simulink model "LBR7_Duobot_ResolvedMotion"  (R2017b)
settings: Solver=ode1  StartTime=0.0  StopTime=12  FixedStep=0.001  RelTol=1e-3
PreLoadFcn:
  | Preload
values from neighbouring files (symbols this model uses):
  joint1_gain = 1    [Preload.m]    (also in PreloadTest.m)
  joint2_gain = 1    [Preload.m]    (also in PreloadTest.m)
  joint3_gain = 1    [Preload.m]    (also in PreloadTest.m)
  joint4_gain = 1    [Preload.m]    (also in PreloadTest.m)
  joint5_gain = 1    [Preload.m]    (also in PreloadTest.m)
  joint6_gain = 1    [Preload.m]    (also in PreloadTest.m)
  joint7_gain = 1    [Preload.m]    (also in PreloadTest.m)
  kuk = SerialLink(L)    [Preload.m]    (also in PreloadTest.m)
undefined symbols (not defined in the file or in its folder): jacky, X, Y, Z
libraries: sm_lib x154, nesl_utility x39
(part 1 of 4)
settings Model: Creator=jrv  LastModifiedBy=mkiri

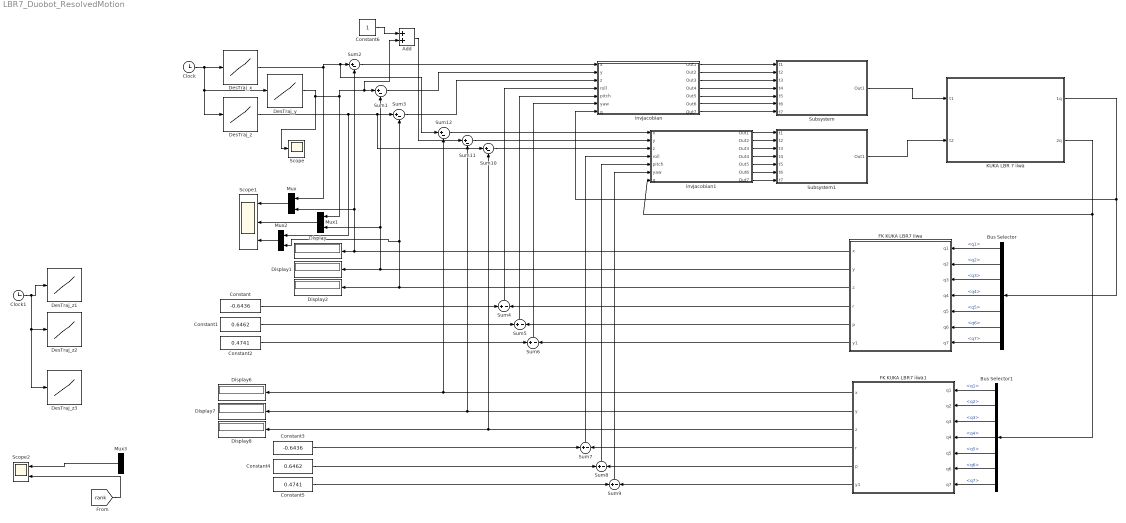
== system LBR7_Duobot_ResolvedMotion ==
  Add : Sum
  Bus Selector : BusSelector  OutputSignals=q1,q2,q3,q4,q5,q6,q7
  Bus Selector1 : BusSelector  OutputSignals=q1,q2,q3,q4,q5,q6,q7
  Clock : Clock
  Clock1 : Clock
  Constant : Constant  Value=-0.6436
  Constant1 : Constant  Value=0.6462
  Constant2 : Constant  Value=0.4741
  Constant3 : Constant  Value=-0.6436
  Constant4 : Constant  Value=0.6462
  Constant5 : Constant  Value=0.4741
  Constant6 : Constant
  DesTraj_x : Lookup_n-D  NumberOfTableDimensions=1  BreakpointsForDimension1=[0 5]  Table=[0.2314 0.2314]  ExtrapMethod=Clip  UseLastTableValue=on  InternalRulePriority=Speed  RndMeth=Simplest  InputSameDT=on
  DesTraj_y : Lookup_n-D  NumberOfTableDimensions=1  BreakpointsForDimension1=[0 12]  Table=[-0.2689 0.0689]  ExtrapMethod=Clip  UseLastTableValue=on  InternalRulePriority=Speed  RndMeth=Simplest  InputSameDT=on
  DesTraj_z : Lookup_n-D  NumberOfTableDimensions=1  BreakpointsForDimension1=[0 3 6 9 12]  Table=[0.9093 0.7093 0.9093 0.7093 0.9093]  InterpMethod=Cubic spline  ExtrapMethod=Clip  UseLastTableValue=on  InternalRulePriority=Speed  RndMeth=Simplest  InputSameDT=on
  DesTraj_z1 : Lookup_n-D  NumberOfTableDimensions=1  BreakpointsForDimension1=[0 1.5]  Table=[-0.6436 0]  ExtrapMethod=Clip  UseLastTableValue=on  InternalRulePriority=Speed  RndMeth=Simplest  InputSameDT=on
  DesTraj_z2 : Lookup_n-D  NumberOfTableDimensions=1  BreakpointsForDimension1=[0 1.5]  Table=[0.6462 0]  ExtrapMethod=Clip  UseLastTableValue=on  InternalRulePriority=Speed  RndMeth=Simplest  InputSameDT=on
  DesTraj_z3 : Lookup_n-D  NumberOfTableDimensions=1  BreakpointsForDimension1=[0 1.5]  Table=[0.4741 0]  ExtrapMethod=Clip  UseLastTableValue=on  InternalRulePriority=Speed  RndMeth=Simplest  InputSameDT=on
  Display{,1..2,6..8} (6 alike) : Display
  FK KUKA LBR7 iiwa : MATLAB Function  TreatAsAtomicUnit=on
  FK KUKA LBR7 iiwa1 : MATLAB Function  TreatAsAtomicUnit=on
  KUKA LBR 7 iiwa : Subsystem
  Mux : Mux  Inputs=2
  Mux1 : Mux  Inputs=2
  Mux2 : Mux  Inputs=2
  Mux3 : Mux  Inputs=3
  Scope : Scope
  Scope1 : Scope  NumInputPorts=3
  Scope2 : Scope  NumInputPorts=2
  Subsystem : Subsystem
  Subsystem1 : Subsystem
  Sum{1..3,10..12} (6 alike) : Sum  Inputs=|+-
  Sum{4..9} (6 alike) : Sum  Inputs=+-
  invJacobian : Subsystem
  invJacobian1 : Subsystem
  wires:
  Subsystem/1(Out1) -> KUKA LBR 7 iiwa/1(t1)
  KUKA LBR 7 iiwa/1(1q) -> invJacobian/7(q), Bus Selector/1
  Bus Selector/3 -> FK KUKA LBR7 iiwa/3(q3)  "<q3>"
  Bus Selector/2 -> FK KUKA LBR7 iiwa/2(q2)  "<q2>"
  Bus Selector/4 -> FK KUKA LBR7 iiwa/4(q4)  "<q4>"
  Bus Selector/1 -> FK KUKA LBR7 iiwa/1(q1)  "<q1>"
  Bus Selector/5 -> FK KUKA LBR7 iiwa/5(q5)  "<q5>"
  Bus Selector/6 -> FK KUKA LBR7 iiwa/6(q6)  "<q6>"
  Bus Selector/7 -> FK KUKA LBR7 iiwa/7(q7)  "<q7>"
  FK KUKA LBR7 iiwa/1(x) -> Mux/2, Sum2/2, Display/1
  FK KUKA LBR7 iiwa/2(y) -> Mux1/2, Sum1/2, Display1/1
  FK KUKA LBR7 iiwa/3(z) -> Mux2/2, Sum3/2, Display2/1
  DesTraj_x/1 -> Mux/1, Sum12/1, Sum2/1
  DesTraj_y/1 -> Scope/1, Mux1/1, Add/2, Sum1/1
  Sum2/1 -> invJacobian/1(x)
  Sum1/1 -> invJacobian/2(y)
  Sum3/1 -> invJacobian/3(z)
  DesTraj_z/1 -> Mux2/1, Sum10/1, Sum3/1
  invJacobian/1(Out1) -> Subsystem/1(t1)
  invJacobian/2(Out2) -> Subsystem/2(t2)
  invJacobian/3(Out3) -> Subsystem/3(t3)
  invJacobian/4(Out4) -> Subsystem/4(t4)
  invJacobian/5(Out5) -> Subsystem/5(t5)
  invJacobian/6(Out6) -> Subsystem/6(t6)
  invJacobian/7(Out7) -> Subsystem/7(t7)
  Clock/1 -> DesTraj_y/1, DesTraj_z/1, DesTraj_x/1
  Mux/1 -> Scope1/1
  Mux1/1 -> Scope1/2
  Mux2/1 -> Scope1/3
  FK KUKA LBR7 iiwa/4(r) -> Sum4/2
  FK KUKA LBR7 iiwa/5(p) -> Sum5/2
  Sum6/1 -> invJacobian/6(yaw)
  Sum4/1 -> invJacobian/4(roll)
  Mux3/1 -> Scope2/1
  [rank] -> Scope2/2
  Clock1/1 -> DesTraj_z3/1, DesTraj_z2/1, DesTraj_z1/1
  invJacobian1/7(Out7) -> Subsystem1/7(t7)
  invJacobian1/6(Out6) -> Subsystem1/6(t6)
  invJacobian1/5(Out5) -> Subsystem1/5(t5)
  invJacobian1/4(Out4) -> Subsystem1/4(t4)
  invJacobian1/3(Out3) -> Subsystem1/3(t3)
  invJacobian1/2(Out2) -> Subsystem1/2(t2)
  invJacobian1/1(Out1) -> Subsystem1/1(t1)
  Subsystem1/1(Out1) -> KUKA LBR 7 iiwa/2(t2)
  Bus Selector1/7 -> FK KUKA LBR7 iiwa1/7(q7)  "<q7>"
  Bus Selector1/6 -> FK KUKA LBR7 iiwa1/6(q6)  "<q6>"
  Bus Selector1/5 -> FK KUKA LBR7 iiwa1/5(q5)  "<q5>"
  Bus Selector1/1 -> FK KUKA LBR7 iiwa1/1(q1)  "<q1>"
  Bus Selector1/4 -> FK KUKA LBR7 iiwa1/4(q4)  "<q4>"
  Bus Selector1/2 -> FK KUKA LBR7 iiwa1/2(q2)  "<q2>"
  Bus Selector1/3 -> FK KUKA LBR7 iiwa1/3(q3)  "<q3>"
  KUKA LBR 7 iiwa/2(2q) -> Bus Selector1/1, invJacobian1/7(q)
  FK KUKA LBR7 iiwa1/1(x) -> Sum12/2, Display6/1
  FK KUKA LBR7 iiwa1/2(y) -> Sum11/2, Display7/1
  FK KUKA LBR7 iiwa1/3(z) -> Display8/1, Sum10/2
  Constant/1 -> Sum4/1
  Constant1/1 -> Sum5/1
  Constant2/1 -> Sum6/1
  FK KUKA LBR7 iiwa/6(y1) -> Sum6/2
  Sum5/1 -> invJacobian/5(pitch)
  Sum8/1 -> invJacobian1/5(pitch)
  FK KUKA LBR7 iiwa1/6(y1) -> Sum9/2
  Constant5/1 -> Sum9/1
  Constant4/1 -> Sum8/1
  Constant3/1 -> Sum7/1
  Sum7/1 -> invJacobian1/4(roll)
  Sum9/1 -> invJacobian1/6(yaw)
  FK KUKA LBR7 iiwa1/5(p) -> Sum8/2
  FK KUKA LBR7 iiwa1/4(r) -> Sum7/2
  Sum10/1 -> invJacobian1/3(z)
  Sum11/1 -> invJacobian1/2(y)
  Sum12/1 -> invJacobian1/1(x)
  Constant6/1 -> Add/1
  Add/1 -> Sum11/1

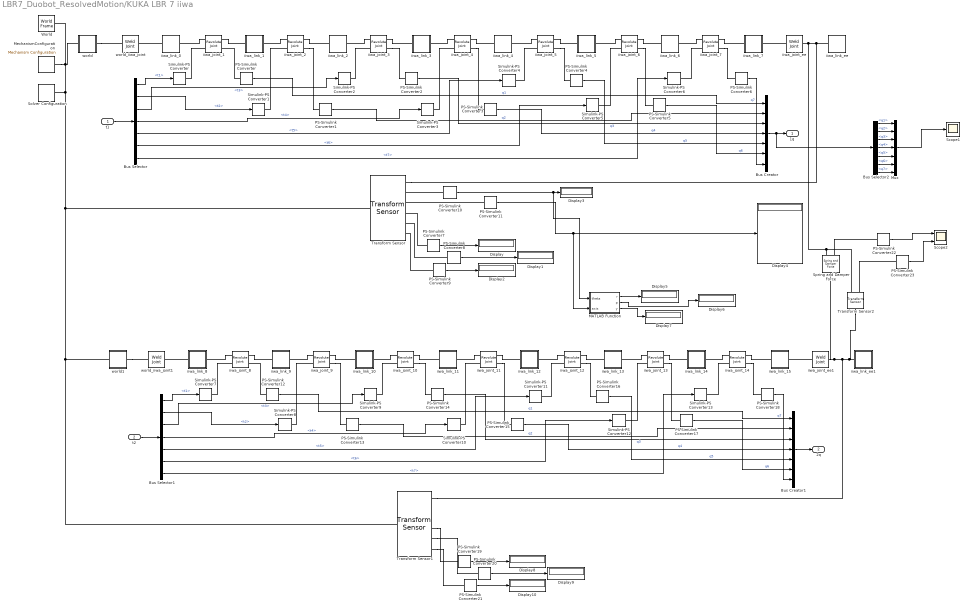
== system LBR7_Duobot_ResolvedMotion/KUKA LBR 7 iiwa ==
  t1 : Inport
  t2 : Inport  Port=2
  Bus Creator : BusCreator  Inputs=7
  Bus Creator1 : BusCreator  Inputs=7
  Bus Selector : BusSelector  OutputSignals=t1,t2,t3,t4,t5,t6,t7
  Bus Selector1 : BusSelector  OutputSignals=t1,t2,t3,t4,t5,t6,t7
  Bus Selector2 : BusSelector  OutputSignals=q1,q2,q3,q4,q5,q6,q7
  Display{,1..10} (11 alike) : Display
  MATLAB Function : MATLAB Function  TreatAsAtomicUnit=on
  MechanismConfiguration : sm_lib/Utilities/Mechanism Configuration  UniformGravity=Constant  GravityVector=[0 0 0]  GravityUnits=m/s^2  LinearizationDelta=0.001
  Mux : Mux  Inputs=7
  PS-Simulink Converter{,1..6,12..18} (14 alike) : nesl_utility/PS-Simulink Converter  PhysicalDomain=network_engine_domain  SubClassName=ps_output  LeftPortType=input  RightPortType=output  PseudoPeriodic=off  Frequencies=[]  Unit=rad  AffineConversion=off
  PS-Simulink Converter{7..11,19..21} (8 alike) : nesl_utility/PS-Simulink Converter  PhysicalDomain=network_engine_domain  SubClassName=ps_output  LeftPortType=input  RightPortType=output  PseudoPeriodic=off  Frequencies=[]  Unit=1  AffineConversion=off
  PS-Simulink Converter22 : nesl_utility/PS-Simulink Converter  PhysicalDomain=network_engine_domain  SubClassName=ps_output  LeftPortType=input  RightPortType=output  PseudoPeriodic=off  Frequencies=[]  Unit=N  AffineConversion=off
  PS-Simulink Converter23 : nesl_utility/PS-Simulink Converter  PhysicalDomain=network_engine_domain  SubClassName=ps_output  LeftPortType=input  RightPortType=output  PseudoPeriodic=off  Frequencies=[]  Unit=m  AffineConversion=off
  Scope1 : Scope
  Scope2 : Scope  NumInputPorts=2
  Simulink-PS Converter{,1..13} (14 alike) : nesl_utility/Simulink-PS Converter  PhysicalDomain=network_engine_domain  SubClassName=ps_input  LeftPortType=input  RightPortType=output  PseudoPeriodic=off  Frequencies=[]  NoiseDistribution=none  NoiseParameters=[]  Unit=N*m  AffineConversion=off  FilteringAndDerivatives=provide  SimscapeFilterOrder=1  InputFilterTimeConstant=0.001  UdotUserProvided=0
  Solver Configuration : nesl_utility/Solver Configuration  PhysicalDomain=network_engine_domain  SubClassName=solver  LeftPortType=input  RightPortType=generic  Accelerate=off  Tones=[]  Harmonics=[]  SimulateNoise=off  Profile=off  UseLocalSampling=off  EnableSwitchedLinearOptims=on  FrequencyDomain=off  UseCCode=off  RelTol=0.001  AbsTol=1e-06  MinStep=1e-09  ToWorkspace=off  RevertToSquareIcSolve=off  NumHomotopyIterations=100  PhasorMode=off  PhasorModeNumHarmonics=1  DoDC=off  ResidualTolerance=1e-09  UseLocalSolver=off  LocalSolverChoice=NE_BACKWARD_EULER_ADVANCER  LocalSolverSampleTime=0.001  DoFixedCost=off  MaxNonlinIter=3  MaxModeIter=2  LinearAlgebra=Sparse  DelaysMemoryBudget=1024  AutomaticFiltering=on  FilteringTimeConstant=0.001
  Spring and Damper Force : sm_lib/Forces and Torques/Spring and Damper Force  NaturalLength=1  NaturalLengthUnits=m  SpringStiffness=200000  SpringStiffnessUnits=N/m  DampingCoefficient=220  DampingCoefficientUnits=N/(m/s)  SenseForce=on
      settings: SourceProductName=Simscape Multibody
  Transform Sensor : sm_lib/Frames and Transforms/Transform Sensor  MeasurementFrame=World  SenseAngle=on  SenseAxis=on  SenseAngle1=off  SenseAngle2=off  SenseAngle3=off  SenseQ=off  SenseR=off  SenseOmegaX=off  SenseOmegaY=off  SenseOmegaZ=off  SenseOmega1=off  SenseOmega2=off  SenseOmega3=off  SenseQDot=off  SenseRDot=off  SenseAlphaX=off  SenseAlphaY=off  SenseAlphaZ=off  SenseAlpha1=off  SenseAlpha2=off  SenseAlpha3=off  SenseQDDot=off  SenseRDDot=off  SenseX=on  SenseY=on  SenseZ=on  SenseRad=off  SenseAzim=off  SenseDist=off  SenseInc=off  SenseXDot=off  SenseYDot=off  SenseZDot=off  SenseRadDot=off  SenseAzimDot=off  SenseDistDot=off  SenseIncDot=off  SenseXDDot=off  SenseYDDot=off  SenseZDDot=off  SenseRadDDot=off  SenseAzimDDot=off  SenseDistDDot=off  SenseIncDDot=off
  Transform Sensor1 : sm_lib/Frames and Transforms/Transform Sensor  MeasurementFrame=World  SenseAngle=on  SenseAxis=on  SenseAngle1=off  SenseAngle2=off  SenseAngle3=off  SenseQ=off  SenseR=off  SenseOmegaX=off  SenseOmegaY=off  SenseOmegaZ=off  SenseOmega1=off  SenseOmega2=off  SenseOmega3=off  SenseQDot=off  SenseRDot=off  SenseAlphaX=off  SenseAlphaY=off  SenseAlphaZ=off  SenseAlpha1=off  SenseAlpha2=off  SenseAlpha3=off  SenseQDDot=off  SenseRDDot=off  SenseX=on  SenseY=on  SenseZ=on  SenseRad=off  SenseAzim=off  SenseDist=off  SenseInc=off  SenseXDot=off  SenseYDot=off  SenseZDot=off  SenseRadDot=off  SenseAzimDot=off  SenseDistDot=off  SenseIncDot=off  SenseXDDot=off  SenseYDDot=off  SenseZDDot=off  SenseRadDDot=off  SenseAzimDDot=off  SenseDistDDot=off  SenseIncDDot=off
  Transform Sensor2 : sm_lib/Frames and Transforms/Transform Sensor  MeasurementFrame=World  SenseAngle=off  SenseAxis=off  SenseAngle1=off  SenseAngle2=off  SenseAngle3=off  SenseQ=off  SenseR=off  SenseOmegaX=off  SenseOmegaY=off  SenseOmegaZ=off  SenseOmega1=off  SenseOmega2=off  SenseOmega3=off  SenseQDot=off  SenseRDot=off  SenseAlphaX=off  SenseAlphaY=off  SenseAlphaZ=off  SenseAlpha1=off  SenseAlpha2=off  SenseAlpha3=off  SenseQDDot=off  SenseRDDot=off  SenseX=off  SenseY=off  SenseZ=off  SenseRad=off  SenseAzim=off  SenseDist=on  SenseInc=off  SenseXDot=off  SenseYDot=off  SenseZDot=off  SenseRadDot=off  SenseAzimDot=off  SenseDistDot=off  SenseIncDot=off  SenseXDDot=off  SenseYDDot=off  SenseZDDot=off  SenseRadDDot=off  SenseAzimDDot=off  SenseDistDDot=off  SenseIncDDot=off
  World : sm_lib/Frames and Transforms/World Frame
  iiwa_joint_1 : sm_lib/Joints/Revolute Joint  SenseConstraintForce=off  SenseConstraintForceX=off  SenseConstraintForceY=off  SenseConstraintForceZ=off  SenseConstraintTorque=off  SenseConstraintTorqueX=off  SenseConstraintTorqueY=off  SenseConstraintTorqueZ=off  SenseTotalForce=off  SenseTotalForceX=off  SenseTotalForceY=off  SenseTotalForceZ=off  SenseTotalTorque=off  SenseTotalTorqueX=off  SenseTotalTorqueY=off  SenseTotalTorqueZ=off  CompositeWrenchDir=FollowerOnBase  CompositeWrenchFrame=BaseFrame  EquilibriumPosition=0  EquilibriumPositionUnits=deg  SpringStiffness=0  SpringStiffnessUnits=N*m/deg  DampingCoefficient=0.5  DampingCoefficientUnits=m^2*kg/s/rad  TorqueActuationMode=InputTorque  MotionActuationMode=ComputedMotion  SensePosition=on  SenseVelocity=off  SenseAcceleration=off  SenseTorqueForce=off  PositionTargetSpecify=on  PositionTargetPriority=High  PositionTargetValue=joint1_initial_deg  PositionTargetValueUnits=deg  VelocityTargetSpecify=off  VelocityTargetPriority=High  VelocityTargetValue=0  VelocityTargetValueUnits=deg/s
  iiwa_joint_10 : sm_lib/Joints/Revolute Joint  SenseConstraintForce=off  SenseConstraintForceX=off  SenseConstraintForceY=off  SenseConstraintForceZ=off  SenseConstraintTorque=off  SenseConstraintTorqueX=off  SenseConstraintTorqueY=off  SenseConstraintTorqueZ=off  SenseTotalForce=off  SenseTotalForceX=off  SenseTotalForceY=off  SenseTotalForceZ=off  SenseTotalTorque=off  SenseTotalTorqueX=off  SenseTotalTorqueY=off  SenseTotalTorqueZ=off  CompositeWrenchDir=FollowerOnBase  CompositeWrenchFrame=BaseFrame  EquilibriumPosition=0  EquilibriumPositionUnits=deg  SpringStiffness=0  SpringStiffnessUnits=N*m/deg  DampingCoefficient=0.5  DampingCoefficientUnits=m^2*kg/s/rad  TorqueActuationMode=InputTorque  MotionActuationMode=ComputedMotion  SensePosition=on  SenseVelocity=off  SenseAcceleration=off  SenseTorqueForce=off  PositionTargetSpecify=on  PositionTargetPriority=High  PositionTargetValue=joint3_initial_deg2  PositionTargetValueUnits=deg  VelocityTargetSpecify=off  VelocityTargetPriority=High  VelocityTargetValue=0  VelocityTargetValueUnits=deg/s
  iiwa_joint_11 : sm_lib/Joints/Revolute Joint  SenseConstraintForce=off  SenseConstraintForceX=off  SenseConstraintForceY=off  SenseConstraintForceZ=off  SenseConstraintTorque=off  SenseConstraintTorqueX=off  SenseConstraintTorqueY=off  SenseConstraintTorqueZ=off  SenseTotalForce=off  SenseTotalForceX=off  SenseTotalForceY=off  SenseTotalForceZ=off  SenseTotalTorque=off  SenseTotalTorqueX=off  SenseTotalTorqueY=off  SenseTotalTorqueZ=off  CompositeWrenchDir=FollowerOnBase  CompositeWrenchFrame=BaseFrame  EquilibriumPosition=0  EquilibriumPositionUnits=deg  SpringStiffness=0  SpringStiffnessUnits=N*m/deg  DampingCoefficient=0.5  DampingCoefficientUnits=m^2*kg/s/rad  TorqueActuationMode=InputTorque  MotionActuationMode=ComputedMotion  SensePosition=on  SenseVelocity=off  SenseAcceleration=off  SenseTorqueForce=off  PositionTargetSpecify=on  PositionTargetPriority=High  PositionTargetValue=joint4_initial_deg2  PositionTargetValueUnits=deg  VelocityTargetSpecify=off  VelocityTargetPriority=High  VelocityTargetValue=0  VelocityTargetValueUnits=deg/s
  iiwa_joint_12 : sm_lib/Joints/Revolute Joint  SenseConstraintForce=off  SenseConstraintForceX=off  SenseConstraintForceY=off  SenseConstraintForceZ=off  SenseConstraintTorque=off  SenseConstraintTorqueX=off  SenseConstraintTorqueY=off  SenseConstraintTorqueZ=off  SenseTotalForce=off  SenseTotalForceX=off  SenseTotalForceY=off  SenseTotalForceZ=off  SenseTotalTorque=off  SenseTotalTorqueX=off  SenseTotalTorqueY=off  SenseTotalTorqueZ=off  CompositeWrenchDir=FollowerOnBase  CompositeWrenchFrame=BaseFrame  EquilibriumPosition=0  EquilibriumPositionUnits=deg  SpringStiffness=0  SpringStiffnessUnits=N*m/deg  DampingCoefficient=0.5  DampingCoefficientUnits=m^2*kg/s/rad  TorqueActuationMode=InputTorque  MotionActuationMode=ComputedMotion  SensePosition=on  SenseVelocity=off  SenseAcceleration=off  SenseTorqueForce=off  PositionTargetSpecify=on  PositionTargetPriority=High  PositionTargetValue=joint5_initial_deg2  PositionTargetValueUnits=deg  VelocityTargetSpecify=off  VelocityTargetPriority=High  VelocityTargetValue=0  VelocityTargetValueUnits=deg/s
  iiwa_joint_13 : sm_lib/Joints/Revolute Joint  SenseConstraintForce=off  SenseConstraintForceX=off  SenseConstraintForceY=off  SenseConstraintForceZ=off  SenseConstraintTorque=off  SenseConstraintTorqueX=off  SenseConstraintTorqueY=off  SenseConstraintTorqueZ=off  SenseTotalForce=off  SenseTotalForceX=off  SenseTotalForceY=off  SenseTotalForceZ=off  SenseTotalTorque=off  SenseTotalTorqueX=off  SenseTotalTorqueY=off  SenseTotalTorqueZ=off  CompositeWrenchDir=FollowerOnBase  CompositeWrenchFrame=BaseFrame  EquilibriumPosition=0  EquilibriumPositionUnits=deg  SpringStiffness=0  SpringStiffnessUnits=N*m/deg  DampingCoefficient=0.5  DampingCoefficientUnits=m^2*kg/s/rad  TorqueActuationMode=InputTorque  MotionActuationMode=ComputedMotion  SensePosition=on  SenseVelocity=off  SenseAcceleration=off  SenseTorqueForce=off  PositionTargetSpecify=on  PositionTargetPriority=High  PositionTargetValue=joint6_initial_deg2  PositionTargetValueUnits=deg  VelocityTargetSpecify=off  VelocityTargetPriority=High  VelocityTargetValue=0  VelocityTargetValueUnits=deg/s
  iiwa_joint_14 : sm_lib/Joints/Revolute Joint  SenseConstraintForce=off  SenseConstraintForceX=off  SenseConstraintForceY=off  SenseConstraintForceZ=off  SenseConstraintTorque=off  SenseConstraintTorqueX=off  SenseConstraintTorqueY=off  SenseConstraintTorqueZ=off  SenseTotalForce=off  SenseTotalForceX=off  SenseTotalForceY=off  SenseTotalForceZ=off  SenseTotalTorque=off  SenseTotalTorqueX=off  SenseTotalTorqueY=off  SenseTotalTorqueZ=off  CompositeWrenchDir=FollowerOnBase  CompositeWrenchFrame=BaseFrame  EquilibriumPosition=0  EquilibriumPositionUnits=deg  SpringStiffness=0  SpringStiffnessUnits=N*m/deg  DampingCoefficient=0.5  DampingCoefficientUnits=m^2*kg/s/rad  TorqueActuationMode=InputTorque  MotionActuationMode=ComputedMotion  SensePosition=on  SenseVelocity=off  SenseAcceleration=off  SenseTorqueForce=off  PositionTargetSpecify=on  PositionTargetPriority=High  PositionTargetValue=joint7_initial_deg2  PositionTargetValueUnits=deg  VelocityTargetSpecify=off  VelocityTargetPriority=High  VelocityTargetValue=0  VelocityTargetValueUnits=deg/s
  iiwa_joint_2 : sm_lib/Joints/Revolute Joint  SenseConstraintForce=off  SenseConstraintForceX=off  SenseConstraintForceY=off  SenseConstraintForceZ=off  SenseConstraintTorque=off  SenseConstraintTorqueX=off  SenseConstraintTorqueY=off  SenseConstraintTorqueZ=off  SenseTotalForce=off  SenseTotalForceX=off  SenseTotalForceY=off  SenseTotalForceZ=off  SenseTotalTorque=off  SenseTotalTorqueX=off  SenseTotalTorqueY=off  SenseTotalTorqueZ=off  CompositeWrenchDir=FollowerOnBase  CompositeWrenchFrame=BaseFrame  EquilibriumPosition=0  EquilibriumPositionUnits=deg  SpringStiffness=0  SpringStiffnessUnits=N*m/deg  DampingCoefficient=0.5  DampingCoefficientUnits=m^2*kg/s/rad  TorqueActuationMode=InputTorque  MotionActuationMode=ComputedMotion  SensePosition=on  SenseVelocity=off  SenseAcceleration=off  SenseTorqueForce=off  PositionTargetSpecify=on  PositionTargetPriority=High  PositionTargetValue=joint2_initial_deg  PositionTargetValueUnits=deg  VelocityTargetSpecify=off  VelocityTargetPriority=High  VelocityTargetValue=0  VelocityTargetValueUnits=deg/s
  iiwa_joint_3 : sm_lib/Joints/Revolute Joint  SenseConstraintForce=off  SenseConstraintForceX=off  SenseConstraintForceY=off  SenseConstraintForceZ=off  SenseConstraintTorque=off  SenseConstraintTorqueX=off  SenseConstraintTorqueY=off  SenseConstraintTorqueZ=off  SenseTotalForce=off  SenseTotalForceX=off  SenseTotalForceY=off  SenseTotalForceZ=off  SenseTotalTorque=off  SenseTotalTorqueX=off  SenseTotalTorqueY=off  SenseTotalTorqueZ=off  CompositeWrenchDir=FollowerOnBase  CompositeWrenchFrame=BaseFrame  EquilibriumPosition=0  EquilibriumPositionUnits=deg  SpringStiffness=0  SpringStiffnessUnits=N*m/deg  DampingCoefficient=0.5  DampingCoefficientUnits=m^2*kg/s/rad  TorqueActuationMode=InputTorque  MotionActuationMode=ComputedMotion  SensePosition=on  SenseVelocity=off  SenseAcceleration=off  SenseTorqueForce=off  PositionTargetSpecify=on  PositionTargetPriority=High  PositionTargetValue=joint3_initial_deg  PositionTargetValueUnits=deg  VelocityTargetSpecify=off  VelocityTargetPriority=High  VelocityTargetValue=0  VelocityTargetValueUnits=deg/s
  iiwa_joint_4 : sm_lib/Joints/Revolute Joint  SenseConstraintForce=off  SenseConstraintForceX=off  SenseConstraintForceY=off  SenseConstraintForceZ=off  SenseConstraintTorque=off  SenseConstraintTorqueX=off  SenseConstraintTorqueY=off  SenseConstraintTorqueZ=off  SenseTotalForce=off  SenseTotalForceX=off  SenseTotalForceY=off  SenseTotalForceZ=off  SenseTotalTorque=off  SenseTotalTorqueX=off  SenseTotalTorqueY=off  SenseTotalTorqueZ=off  CompositeWrenchDir=FollowerOnBase  CompositeWrenchFrame=BaseFrame  EquilibriumPosition=0  EquilibriumPositionUnits=deg  SpringStiffness=0  SpringStiffnessUnits=N*m/deg  DampingCoefficient=0.5  DampingCoefficientUnits=m^2*kg/s/rad  TorqueActuationMode=InputTorque  MotionActuationMode=ComputedMotion  SensePosition=on  SenseVelocity=off  SenseAcceleration=off  SenseTorqueForce=off  PositionTargetSpecify=on  PositionTargetPriority=High  PositionTargetValue=joint4_initial_deg  PositionTargetValueUnits=deg  VelocityTargetSpecify=off  VelocityTargetPriority=High  VelocityTargetValue=0  VelocityTargetValueUnits=deg/s
  iiwa_joint_5 : sm_lib/Joints/Revolute Joint  SenseConstraintForce=off  SenseConstraintForceX=off  SenseConstraintForceY=off  SenseConstraintForceZ=off  SenseConstraintTorque=off  SenseConstraintTorqueX=off  SenseConstraintTorqueY=off  SenseConstraintTorqueZ=off  SenseTotalForce=off  SenseTotalForceX=off  SenseTotalForceY=off  SenseTotalForceZ=off  SenseTotalTorque=off  SenseTotalTorqueX=off  SenseTotalTorqueY=off  SenseTotalTorqueZ=off  CompositeWrenchDir=FollowerOnBase  CompositeWrenchFrame=BaseFrame  EquilibriumPosition=0  EquilibriumPositionUnits=deg  SpringStiffness=0  SpringStiffnessUnits=N*m/deg  DampingCoefficient=0.5  DampingCoefficientUnits=m^2*kg/s/rad  TorqueActuationMode=InputTorque  MotionActuationMode=ComputedMotion  SensePosition=on  SenseVelocity=off  SenseAcceleration=off  SenseTorqueForce=off  PositionTargetSpecify=on  PositionTargetPriority=High  PositionTargetValue=joint5_initial_deg  PositionTargetValueUnits=deg  VelocityTargetSpecify=off  VelocityTargetPriority=High  VelocityTargetValue=0  VelocityTargetValueUnits=deg/s
  iiwa_joint_6 : sm_lib/Joints/Revolute Joint  SenseConstraintForce=off  SenseConstraintForceX=off  SenseConstraintForceY=off  SenseConstraintForceZ=off  SenseConstraintTorque=off  SenseConstraintTorqueX=off  SenseConstraintTorqueY=off  SenseConstraintTorqueZ=off  SenseTotalForce=off  SenseTotalForceX=off  SenseTotalForceY=off  SenseTotalForceZ=off  SenseTotalTorque=off  SenseTotalTorqueX=off  SenseTotalTorqueY=off  SenseTotalTorqueZ=off  CompositeWrenchDir=FollowerOnBase  CompositeWrenchFrame=BaseFrame  EquilibriumPosition=0  EquilibriumPositionUnits=deg  SpringStiffness=0  SpringStiffnessUnits=N*m/deg  DampingCoefficient=0.5  DampingCoefficientUnits=m^2*kg/s/rad  TorqueActuationMode=InputTorque  MotionActuationMode=ComputedMotion  SensePosition=on  SenseVelocity=off  SenseAcceleration=off  SenseTorqueForce=off  PositionTargetSpecify=on  PositionTargetPriority=High  PositionTargetValue=joint6_initial_deg  PositionTargetValueUnits=deg  VelocityTargetSpecify=off  VelocityTargetPriority=High  VelocityTargetValue=0  VelocityTargetValueUnits=deg/s
  iiwa_joint_7 : sm_lib/Joints/Revolute Joint  SenseConstraintForce=off  SenseConstraintForceX=off  SenseConstraintForceY=off  SenseConstraintForceZ=off  SenseConstraintTorque=off  SenseConstraintTorqueX=off  SenseConstraintTorqueY=off  SenseConstraintTorqueZ=off  SenseTotalForce=off  SenseTotalForceX=off  SenseTotalForceY=off  SenseTotalForceZ=off  SenseTotalTorque=off  SenseTotalTorqueX=off  SenseTotalTorqueY=off  SenseTotalTorqueZ=off  CompositeWrenchDir=FollowerOnBase  CompositeWrenchFrame=BaseFrame  EquilibriumPosition=0  EquilibriumPositionUnits=deg  SpringStiffness=0  SpringStiffnessUnits=N*m/deg  DampingCoefficient=0.5  DampingCoefficientUnits=m^2*kg/s/rad  TorqueActuationMode=InputTorque  MotionActuationMode=ComputedMotion  SensePosition=on  SenseVelocity=off  SenseAcceleration=off  SenseTorqueForce=off  PositionTargetSpecify=on  PositionTargetPriority=High  PositionTargetValue=joint7_initial_deg  PositionTargetValueUnits=deg  VelocityTargetSpecify=off  VelocityTargetPriority=High  VelocityTargetValue=0  VelocityTargetValueUnits=deg/s
  iiwa_joint_8 : sm_lib/Joints/Revolute Joint  SenseConstraintForce=off  SenseConstraintForceX=off  SenseConstraintForceY=off  SenseConstraintForceZ=off  SenseConstraintTorque=off  SenseConstraintTorqueX=off  SenseConstraintTorqueY=off  SenseConstraintTorqueZ=off  SenseTotalForce=off  SenseTotalForceX=off  SenseTotalForceY=off  SenseTotalForceZ=off  SenseTotalTorque=off  SenseTotalTorqueX=off  SenseTotalTorqueY=off  SenseTotalTorqueZ=off  CompositeWrenchDir=FollowerOnBase  CompositeWrenchFrame=BaseFrame  EquilibriumPosition=0  EquilibriumPositionUnits=deg  SpringStiffness=0  SpringStiffnessUnits=N*m/deg  DampingCoefficient=0.5  DampingCoefficientUnits=m^2*kg/s/rad  TorqueActuationMode=InputTorque  MotionActuationMode=ComputedMotion  SensePosition=on  SenseVelocity=off  SenseAcceleration=off  SenseTorqueForce=off  PositionTargetSpecify=on  PositionTargetPriority=High  PositionTargetValue=joint1_initial_deg2  PositionTargetValueUnits=deg  VelocityTargetSpecify=off  VelocityTargetPriority=High  VelocityTargetValue=0  VelocityTargetValueUnits=deg/s
  iiwa_joint_9 : sm_lib/Joints/Revolute Joint  SenseConstraintForce=off  SenseConstraintForceX=off  SenseConstraintForceY=off  SenseConstraintForceZ=off  SenseConstraintTorque=off  SenseConstraintTorqueX=off  SenseConstraintTorqueY=off  SenseConstraintTorqueZ=off  SenseTotalForce=off  SenseTotalForceX=off  SenseTotalForceY=off  SenseTotalForceZ=off  SenseTotalTorque=off  SenseTotalTorqueX=off  SenseTotalTorqueY=off  SenseTotalTorqueZ=off  CompositeWrenchDir=FollowerOnBase  CompositeWrenchFrame=BaseFrame  EquilibriumPosition=0  EquilibriumPositionUnits=deg  SpringStiffness=0  SpringStiffnessUnits=N*m/deg  DampingCoefficient=0.5  DampingCoefficientUnits=m^2*kg/s/rad  TorqueActuationMode=InputTorque  MotionActuationMode=ComputedMotion  SensePosition=on  SenseVelocity=off  SenseAcceleration=off  SenseTorqueForce=off  PositionTargetSpecify=on  PositionTargetPriority=High  PositionTargetValue=joint2_initial_deg2  PositionTargetValueUnits=deg  VelocityTargetSpecify=off  VelocityTargetPriority=High  VelocityTargetValue=0  VelocityTargetValueUnits=deg/s
  iiwa_joint_ee : sm_lib/Joints/Weld Joint  SenseConstraintForce=off  SenseConstraintForceX=off  SenseConstraintForceY=off  SenseConstraintForceZ=off  SenseConstraintTorque=off  SenseConstraintTorqueX=off  SenseConstraintTorqueY=off  SenseConstraintTorqueZ=off  SenseTotalForce=off  SenseTotalForceX=off  SenseTotalForceY=off  SenseTotalForceZ=off  SenseTotalTorque=off  SenseTotalTorqueX=off  SenseTotalTorqueY=off  SenseTotalTorqueZ=off  CompositeWrenchDir=FollowerOnBase  CompositeWrenchFrame=BaseFrame
  iiwa_joint_ee1 : sm_lib/Joints/Weld Joint  SenseConstraintForce=off  SenseConstraintForceX=off  SenseConstraintForceY=off  SenseConstraintForceZ=off  SenseConstraintTorque=off  SenseConstraintTorqueX=off  SenseConstraintTorqueY=off  SenseConstraintTorqueZ=off  SenseTotalForce=off  SenseTotalForceX=off  SenseTotalForceY=off  SenseTotalForceZ=off  SenseTotalTorque=off  SenseTotalTorqueX=off  SenseTotalTorqueY=off  SenseTotalTorqueZ=off  CompositeWrenchDir=FollowerOnBase  CompositeWrenchFrame=BaseFrame
  iiwa_link_0 : Subsystem
  iiwa_link_1 : Subsystem
  iiwa_link_10 : Subsystem
  iiwa_link_11 : Subsystem
  iiwa_link_12 : Subsystem
  iiwa_link_13 : Subsystem
  iiwa_link_14 : Subsystem
  iiwa_link_15 : Subsystem
  iiwa_link_2 : Subsystem
  iiwa_link_3 : Subsystem
  iiwa_link_4 : Subsystem
  iiwa_link_5 : Subsystem
  iiwa_link_6 : Subsystem
  iiwa_link_7 : Subsystem
  iiwa_link_8 : Subsystem
  iiwa_link_9 : Subsystem
  iiwa_link_ee : Subsystem
  iiwa_link_ee1 : Subsystem
  world : Subsystem
  world1 : Subsystem
  world_iiwa_joint : sm_lib/Joints/Weld Joint  SenseConstraintForce=off  SenseConstraintForceX=off  SenseConstraintForceY=off  SenseConstraintForceZ=off  SenseConstraintTorque=off  SenseConstraintTorqueX=off  SenseConstraintTorqueY=off  SenseConstraintTorqueZ=off  SenseTotalForce=off  SenseTotalForceX=off  SenseTotalForceY=off  SenseTotalForceZ=off  SenseTotalTorque=off  SenseTotalTorqueX=off  SenseTotalTorqueY=off  SenseTotalTorqueZ=off  CompositeWrenchDir=FollowerOnBase  CompositeWrenchFrame=BaseFrame
  world_iiwa_joint1 : sm_lib/Joints/Weld Joint  SenseConstraintForce=off  SenseConstraintForceX=off  SenseConstraintForceY=off  SenseConstraintForceZ=off  SenseConstraintTorque=off  SenseConstraintTorqueX=off  SenseConstraintTorqueY=off  SenseConstraintTorqueZ=off  SenseTotalForce=off  SenseTotalForceX=off  SenseTotalForceY=off  SenseTotalForceZ=off  SenseTotalTorque=off  SenseTotalTorqueX=off  SenseTotalTorqueY=off  SenseTotalTorqueZ=off  CompositeWrenchDir=FollowerOnBase  CompositeWrenchFrame=BaseFrame
  1q : Outport
  2q : Outport  Port=2
  wires:
  PS-Simulink Converter7/1 -> Display/1
  PS-Simulink Converter9/1 -> Display2/1
  PS-Simulink Converter8/1 -> Display1/1
  PS-Simulink Converter/1 -> Bus Creator/1  "q1"
  PS-Simulink Converter1/1 -> Bus Creator/2  "q2"
  PS-Simulink Converter2/1 -> Bus Creator/3  "q3"
  PS-Simulink Converter3/1 -> Bus Creator/4  "q4"
  PS-Simulink Converter4/1 -> Bus Creator/5  "q5"
  PS-Simulink Converter5/1 -> Bus Creator/6  "q6"
  PS-Simulink Converter6/1 -> Bus Creator/7  "q7"
  t1/1 -> Bus Selector/1
  Bus Selector/1 -> Simulink-PS Converter/1  "<t1>"
  Bus Selector/2 -> Simulink-PS Converter1/1  "<t2>"
  Bus Selector/3 -> Simulink-PS Converter2/1  "<t3>"
  Bus Selector/4 -> Simulink-PS Converter3/1  "<t4>"
  Bus Selector/5 -> Simulink-PS Converter4/1  "<t5>"
  Bus Selector/6 -> Simulink-PS Converter5/1  "<t6>"
  Bus Selector/7 -> Simulink-PS Converter6/1  "<t7>"
  PS-Simulink Converter10/1 -> MATLAB Function/1(theta), Display3/1
  PS-Simulink Converter11/1 -> MATLAB Function/2(axis), Display4/1
  MATLAB Function/1(r) -> Display5/1
  MATLAB Function/3(y) -> Display7/1
  MATLAB Function/2(p) -> Display6/1
  Bus Selector1/7 -> Simulink-PS Converter13/1  "<t7>"
  Bus Selector1/6 -> Simulink-PS Converter12/1  "<t6>"
  Bus Selector1/5 -> Simulink-PS Converter11/1  "<t5>"
  Bus Selector1/4 -> Simulink-PS Converter10/1  "<t4>"
  Bus Selector1/3 -> Simulink-PS Converter9/1  "<t3>"
  Bus Selector1/2 -> Simulink-PS Converter8/1  "<t2>"
  Bus Selector1/1 -> Simulink-PS Converter7/1  "<t1>"
  t2/1 -> Bus Selector1/1
  Bus Creator1/1 -> 2q/1
  PS-Simulink Converter18/1 -> Bus Creator1/7  "q7"
  PS-Simulink Converter17/1 -> Bus Creator1/6  "q6"
  PS-Simulink Converter16/1 -> Bus Creator1/5  "q5"
  PS-Simulink Converter15/1 -> Bus Creator1/4  "q4"
  PS-Simulink Converter14/1 -> Bus Creator1/3  "q3"
  PS-Simulink Converter13/1 -> Bus Creator1/2  "q2"
  PS-Simulink Converter12/1 -> Bus Creator1/1  "q1"
  PS-Simulink Converter20/1 -> Display9/1
  PS-Simulink Converter21/1 -> Display10/1
  PS-Simulink Converter19/1 -> Display8/1
  PS-Simulink Converter22/1 -> Scope2/1
  PS-Simulink Converter23/1 -> Scope2/2
  Bus Creator/1 -> Bus Selector2/1, 1q/1
  Bus Selector2/1 -> Mux/1  "<q1>"
  Mux/1 -> Scope1/1
  Bus Selector2/6 -> Mux/6  "<q6>"
  Bus Selector2/2 -> Mux/2  "<q2>"
  Bus Selector2/3 -> Mux/3  "<q3>"
  Bus Selector2/5 -> Mux/5  "<q5>"
  Bus Selector2/7 -> Mux/7  "<q7>"
  Bus Selector2/4 -> Mux/4  "<q4>"
  connections:
  Simulink-PS Converter/RConn1 -- iiwa_joint_1/LConn2
  iiwa_joint_5/RConn2 -- PS-Simulink Converter4/LConn1
  iiwa_joint_5/LConn2 -- Simulink-PS Converter4/RConn1
  PS-Simulink Converter/LConn1 -- iiwa_joint_1/RConn2
  iiwa_joint_2/LConn2 -- Simulink-PS Converter1/RConn1
  iiwa_joint_2/RConn2 -- PS-Simulink Converter1/LConn1
  iiwa_joint_6/RConn2 -- PS-Simulink Converter5/LConn1
  iiwa_joint_6/LConn2 -- Simulink-PS Converter5/RConn1
  iiwa_joint_7/RConn2 -- PS-Simulink Converter6/LConn1
  iiwa_joint_7/LConn2 -- Simulink-PS Converter6/RConn1
  iiwa_joint_1/LConn1 -- iiwa_link_0/RConn1
  iiwa_joint_ee/LConn1 -- iiwa_link_7/RConn1
  iiwa_joint_2/RConn1 -- iiwa_link_2/LConn1
  iiwa_joint_7/RConn1 -- iiwa_link_7/LConn1
  iiwa_link_0/LConn1 -- world_iiwa_joint/RConn1
  iiwa_joint_6/RConn1 -- iiwa_link_6/LConn1
  world/RConn1 -- world_iiwa_joint/LConn1
  iiwa_joint_3/RConn1 -- iiwa_link_3/LConn1
  iiwa_joint_4/LConn1 -- iiwa_link_3/RConn1
  World/RConn1 -- Transform Sensor1/LConn1 -- world1/LConn1 -- Transform Sensor/LConn1 -- Solver Configuration/RConn1 -- MechanismConfiguration/RConn1 -- world/LConn1
  iiwa_joint_6/LConn1 -- iiwa_link_5/RConn1
  iiwa_joint_3/LConn1 -- iiwa_link_2/RConn1
  iiwa_joint_5/RConn1 -- iiwa_link_5/LConn1
  iiwa_joint_5/LConn1 -- iiwa_link_4/RConn1
  iiwa_joint_ee/RConn1 -- Transform Sensor2/RConn1 -- Spring and Damper Force/RConn1 -- iiwa_link_ee/LConn1 -- Transform Sensor/RConn1
  iiwa_joint_2/LConn1 -- iiwa_link_1/RConn1
  iiwa_joint_7/LConn1 -- iiwa_link_6/RConn1
  iiwa_joint_1/RConn1 -- iiwa_link_1/LConn1
  iiwa_joint_4/RConn1 -- iiwa_link_4/LConn1
  iiwa_joint_4/LConn2 -- Simulink-PS Converter3/RConn1
  iiwa_joint_4/RConn2 -- PS-Simulink Converter3/LConn1
  iiwa_joint_3/RConn2 -- PS-Simulink Converter2/LConn1
  iiwa_joint_3/LConn2 -- Simulink-PS Converter2/RConn1
  PS-Simulink Converter10/LConn1 -- Transform Sensor/RConn2
  PS-Simulink Converter11/LConn1 -- Transform Sensor/RConn3
  PS-Simulink Converter7/LConn1 -- Transform Sensor/RConn4
  PS-Simulink Converter9/LConn1 -- Transform Sensor/RConn6
  PS-Simulink Converter8/LConn1 -- Transform Sensor/RConn5
  iiwa_joint_ee1/RConn1 -- Transform Sensor2/LConn1 -- iiwa_link_ee1/LConn1 -- Transform Sensor1/RConn1 -- Spring and Damper Force/LConn1
  iiwa_joint_10/RConn2 -- PS-Simulink Converter14/LConn1
  iiwa_joint_11/RConn2 -- PS-Simulink Converter15/LConn1
  iiwa_joint_11/RConn1 -- iiwa_link_12/LConn1
  iiwa_joint_14/LConn1 -- iiwa_link_14/RConn1
  iiwa_joint_12/LConn1 -- iiwa_link_12/RConn1
  iiwa_joint_10/LConn1 -- iiwa_link_10/RConn1
  iiwa_joint_12/RConn1 -- iiwa_link_13/LConn1
  iiwa_joint_13/LConn1 -- iiwa_link_13/RConn1
  iiwa_joint_11/LConn1 -- iiwa_link_11/RConn1
  iiwa_joint_10/RConn1 -- iiwa_link_11/LConn1
  iiwa_joint_9/LConn1 -- iiwa_link_9/RConn1
  world1/RConn1 -- world_iiwa_joint1/LConn1
  iiwa_joint_13/RConn1 -- iiwa_link_14/LConn1
  iiwa_joint_14/RConn1 -- iiwa_link_15/LConn1
  iiwa_joint_9/RConn1 -- iiwa_link_10/LConn1
  iiwa_joint_11/LConn2 -- Simulink-PS Converter10/RConn1
  iiwa_joint_ee1/LConn1 -- iiwa_link_15/RConn1
  iiwa_joint_14/LConn2 -- Simulink-PS Converter13/RConn1
  iiwa_joint_8/LConn1 -- iiwa_link_8/RConn1
  iiwa_joint_14/RConn2 -- PS-Simulink Converter18/LConn1
  iiwa_joint_13/RConn2 -- PS-Simulink Converter17/LConn1
  iiwa_link_8/LConn1 -- world_iiwa_joint1/RConn1
  iiwa_joint_13/LConn2 -- Simulink-PS Converter12/RConn1
  iiwa_joint_9/RConn2 -- PS-Simulink Converter13/LConn1
  iiwa_joint_8/RConn1 -- iiwa_link_9/LConn1
  iiwa_joint_12/LConn2 -- Simulink-PS Converter11/RConn1
  iiwa_joint_10/LConn2 -- Simulink-PS Converter9/RConn1
  iiwa_joint_12/RConn2 -- PS-Simulink Converter16/LConn1
  iiwa_joint_9/LConn2 -- Simulink-PS Converter8/RConn1
  Simulink-PS Converter7/RConn1 -- iiwa_joint_8/LConn2
  PS-Simulink Converter12/LConn1 -- iiwa_joint_8/RConn2
  Transform Sensor1/RConn5 -- PS-Simulink Converter20/LConn1
  Transform Sensor1/RConn6 -- PS-Simulink Converter21/LConn1
  Transform Sensor1/RConn4 -- PS-Simulink Converter19/LConn1
  PS-Simulink Converter22/LConn1 -- Spring and Damper Force/RConn2
  PS-Simulink Converter23/LConn1 -- Transform Sensor2/RConn2

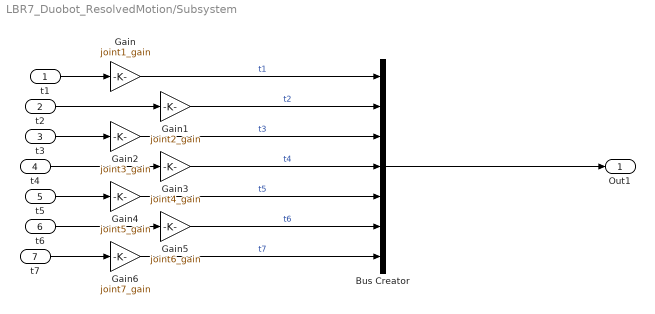
== system LBR7_Duobot_ResolvedMotion/Subsystem ==
  t1 : Inport
  t2 : Inport  Port=2
  t3 : Inport  Port=3
  t4 : Inport  Port=4
  t5 : Inport  Port=5
  t6 : Inport  Port=6
  t7 : Inport  Port=7
  Bus Creator : BusCreator  Inputs=7
  Gain : Gain  Gain=joint1_gain
  Gain1 : Gain  Gain=joint2_gain
  Gain2 : Gain  Gain=joint3_gain
  Gain3 : Gain  Gain=joint4_gain
  Gain4 : Gain  Gain=joint5_gain
  Gain5 : Gain  Gain=joint6_gain
  Gain6 : Gain  Gain=joint7_gain
  Out1 : Outport
  wires:
  Bus Creator/1 -> Out1/1
  t6/1 -> Gain5/1
  t5/1 -> Gain4/1
  t2/1 -> Gain1/1
  t1/1 -> Gain/1
  t7/1 -> Gain6/1
  t4/1 -> Gain3/1
  t3/1 -> Gain2/1
  Gain/1 -> Bus Creator/1  "t1"
  Gain1/1 -> Bus Creator/2  "t2"
  Gain2/1 -> Bus Creator/3  "t3"
  Gain3/1 -> Bus Creator/4  "t4"
  Gain4/1 -> Bus Creator/5  "t5"
  Gain5/1 -> Bus Creator/6  "t6"
  Gain6/1 -> Bus Creator/7  "t7"

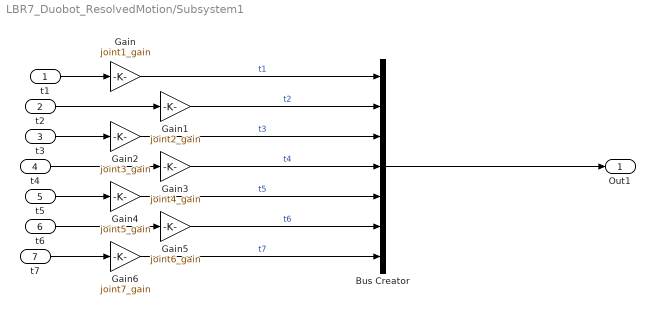
== system LBR7_Duobot_ResolvedMotion/Subsystem1 ==
  t1 : Inport
  t2 : Inport  Port=2
  t3 : Inport  Port=3
  t4 : Inport  Port=4
  t5 : Inport  Port=5
  t6 : Inport  Port=6
  t7 : Inport  Port=7
  Bus Creator : BusCreator  Inputs=7
  Gain : Gain  Gain=joint1_gain
  Gain1 : Gain  Gain=joint2_gain
  Gain2 : Gain  Gain=joint3_gain
  Gain3 : Gain  Gain=joint4_gain
  Gain4 : Gain  Gain=joint5_gain
  Gain5 : Gain  Gain=joint6_gain
  Gain6 : Gain  Gain=joint7_gain
  Out1 : Outport
  wires:
  Gain6/1 -> Bus Creator/7  "t7"
  Gain5/1 -> Bus Creator/6  "t6"
  Gain4/1 -> Bus Creator/5  "t5"
  Gain3/1 -> Bus Creator/4  "t4"
  Gain2/1 -> Bus Creator/3  "t3"
  Gain1/1 -> Bus Creator/2  "t2"
  Gain/1 -> Bus Creator/1  "t1"
  t3/1 -> Gain2/1
  t4/1 -> Gain3/1
  t7/1 -> Gain6/1
  t1/1 -> Gain/1
  t2/1 -> Gain1/1
  t5/1 -> Gain4/1
  t6/1 -> Gain5/1
  Bus Creator/1 -> Out1/1

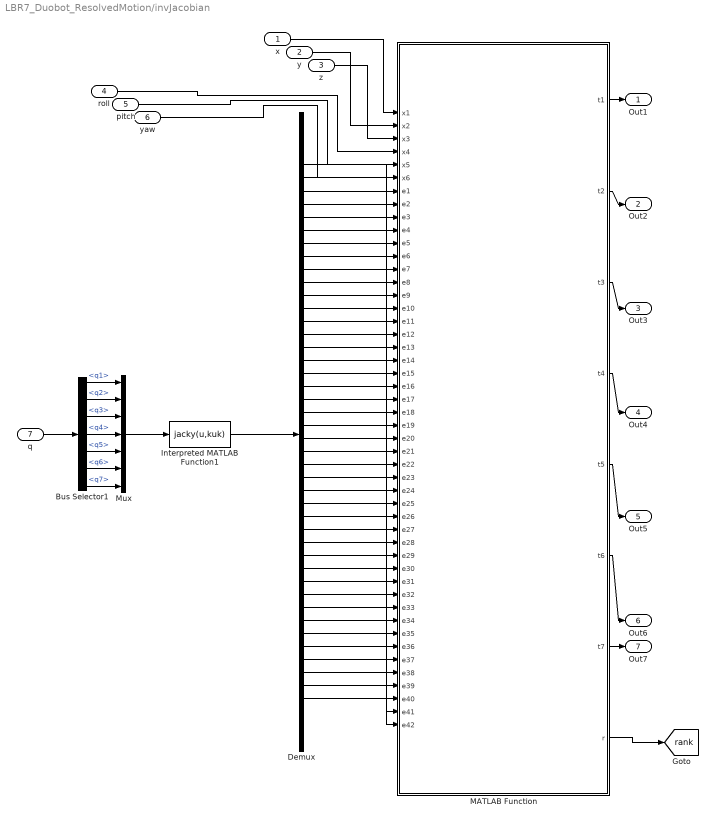
== system LBR7_Duobot_ResolvedMotion/invJacobian ==
  x : Inport
  y : Inport  Port=2
  z : Inport  Port=3
  roll : Inport  Port=4
  pitch : Inport  Port=5
  yaw : Inport  Port=6
  q : Inport  Port=7
  Bus Selector1 : BusSelector  OutputSignals=q1,q2,q3,q4,q5,q6,q7
  Demux : Demux  Outputs=42
  Interpreted MATLAB Function1 : MATLABFcn  MATLABFcn=jacky(u,kuk)
  MATLAB Function : MATLAB Function  TreatAsAtomicUnit=on
  Mux : Mux  Inputs=7
  Out1 : Outport
  Out2 : Outport  Port=2
  Out3 : Outport  Port=3
  Out4 : Outport  Port=4
  Out5 : Outport  Port=5
  Out6 : Outport  Port=6
  Out7 : Outport  Port=7
  tag scope: rank=global
  wires:
  x/1 -> MATLAB Function/1(x1)
  MATLAB Function/2(t2) -> Out2/1
  MATLAB Function/3(t3) -> Out3/1
  y/1 -> MATLAB Function/2(x2)
  MATLAB Function/1(t1) -> Out1/1
  MATLAB Function/4(t4) -> Out4/1
  MATLAB Function/5(t5) -> Out5/1
  z/1 -> MATLAB Function/3(x3)
  MATLAB Function/7(t7) -> Out7/1
  MATLAB Function/6(t6) -> Out6/1
  Interpreted MATLAB Function1/1 -> Demux/1
  Demux/17 -> MATLAB Function/23(e17)
  Demux/16 -> MATLAB Function/22(e16)
  Demux/15 -> MATLAB Function/21(e15)
  Demux/19 -> MATLAB Function/25(e19)
  Demux/14 -> MATLAB Function/20(e14)
  Demux/13 -> MATLAB Function/19(e13)
  Demux/18 -> MATLAB Function/24(e18)
  Demux/20 -> MATLAB Function/26(e20)
  Demux/21 -> MATLAB Function/27(e21)
  Demux/12 -> MATLAB Function/18(e12)
  Demux/6 -> MATLAB Function/12(e6)
  Demux/28 -> MATLAB Function/34(e28)
  Demux/23 -> MATLAB Function/29(e23)
  Demux/5 -> MATLAB Function/11(e5)
  Demux/25 -> MATLAB Function/31(e25)
  Demux/22 -> MATLAB Function/28(e22)
  Demux/9 -> MATLAB Function/15(e9)
  Demux/10 -> MATLAB Function/16(e10)
  Demux/7 -> MATLAB Function/13(e7)
  Demux/11 -> MATLAB Function/17(e11)
  Demux/8 -> MATLAB Function/14(e8)
  Demux/27 -> MATLAB Function/33(e27)
  Demux/26 -> MATLAB Function/32(e26)
  Demux/24 -> MATLAB Function/30(e24)
  Demux/3 -> MATLAB Function/9(e3)
  Demux/38 -> MATLAB Function/44(e38)
  Demux/33 -> MATLAB Function/39(e33)
  Demux/39 -> MATLAB Function/45(e39)
  Demux/36 -> MATLAB Function/42(e36)
  Demux/41 -> MATLAB Function/47(e41)
  Demux/42 -> MATLAB Function/48(e42)
  Demux/40 -> MATLAB Function/46(e40)
  Demux/34 -> MATLAB Function/40(e34)
  Demux/31 -> MATLAB Function/37(e31)
  Demux/30 -> MATLAB Function/36(e30)
  Demux/2 -> MATLAB Function/8(e2)
  Demux/4 -> MATLAB Function/10(e4)
  Demux/32 -> MATLAB Function/38(e32)
  Demux/1 -> MATLAB Function/7(e1)
  Demux/35 -> MATLAB Function/41(e35)
  Demux/37 -> MATLAB Function/43(e37)
  Demux/29 -> MATLAB Function/35(e29)
  q/1 -> Bus Selector1/1
  Bus Selector1/3 -> Mux/3  "<q3>"
  Bus Selector1/2 -> Mux/2  "<q2>"
  Bus Selector1/4 -> Mux/4  "<q4>"
  Bus Selector1/1 -> Mux/1  "<q1>"
  Bus Selector1/5 -> Mux/5  "<q5>"
  Bus Selector1/6 -> Mux/6  "<q6>"
  Bus Selector1/7 -> Mux/7  "<q7>"
  Mux/1 -> Interpreted MATLAB Function1/1
  yaw/1 -> MATLAB Function/6(x6)
  pitch/1 -> MATLAB Function/5(x5)
  roll/1 -> MATLAB Function/4(x4)
  MATLAB Function/8(r) -> [rank]

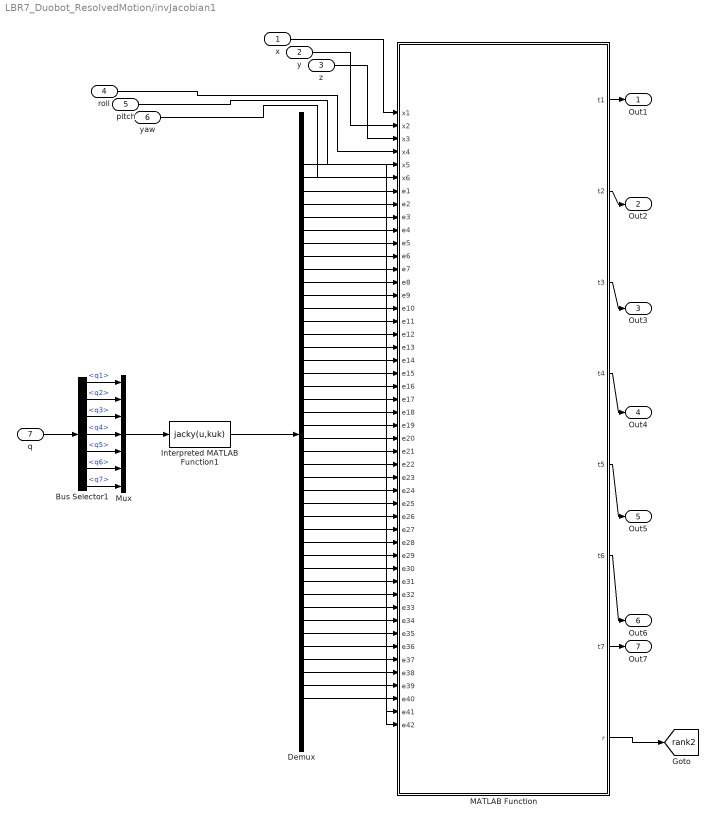
== system LBR7_Duobot_ResolvedMotion/invJacobian1 ==
  x : Inport
  y : Inport  Port=2
  z : Inport  Port=3
  roll : Inport  Port=4
  pitch : Inport  Port=5
  yaw : Inport  Port=6
  q : Inport  Port=7
  Bus Selector1 : BusSelector  OutputSignals=q1,q2,q3,q4,q5,q6,q7
  Demux : Demux  Outputs=42
  Interpreted MATLAB Function1 : MATLABFcn  MATLABFcn=jacky(u,kuk)
  MATLAB Function : MATLAB Function  TreatAsAtomicUnit=on
  Mux : Mux  Inputs=7
  Out1 : Outport
  Out2 : Outport  Port=2
  Out3 : Outport  Port=3
  Out4 : Outport  Port=4
  Out5 : Outport  Port=5
  Out6 : Outport  Port=6
  Out7 : Outport  Port=7
  tag scope: rank2=global
  wires:
  MATLAB Function/8(r) -> [rank2]
  roll/1 -> MATLAB Function/4(x4)
  pitch/1 -> MATLAB Function/5(x5)
  yaw/1 -> MATLAB Function/6(x6)
  Mux/1 -> Interpreted MATLAB Function1/1
  Bus Selector1/7 -> Mux/7  "<q7>"
  Bus Selector1/6 -> Mux/6  "<q6>"
  Bus Selector1/5 -> Mux/5  "<q5>"
  Bus Selector1/1 -> Mux/1  "<q1>"
  Bus Selector1/4 -> Mux/4  "<q4>"
  Bus Selector1/2 -> Mux/2  "<q2>"
  Bus Selector1/3 -> Mux/3  "<q3>"
  q/1 -> Bus Selector1/1
  Demux/29 -> MATLAB Function/35(e29)
  Demux/37 -> MATLAB Function/43(e37)
  Demux/35 -> MATLAB Function/41(e35)
  Demux/1 -> MATLAB Function/7(e1)
  Demux/32 -> MATLAB Function/38(e32)
  Demux/4 -> MATLAB Function/10(e4)
  Demux/2 -> MATLAB Function/8(e2)
  Demux/30 -> MATLAB Function/36(e30)
  Demux/31 -> MATLAB Function/37(e31)
  Demux/34 -> MATLAB Function/40(e34)
  Demux/40 -> MATLAB Function/46(e40)
  Demux/42 -> MATLAB Function/48(e42)
  Demux/41 -> MATLAB Function/47(e41)
  Demux/36 -> MATLAB Function/42(e36)
  Demux/39 -> MATLAB Function/45(e39)
  Demux/33 -> MATLAB Function/39(e33)
  Demux/38 -> MATLAB Function/44(e38)
  Demux/3 -> MATLAB Function/9(e3)
  Demux/24 -> MATLAB Function/30(e24)
  Demux/26 -> MATLAB Function/32(e26)
  Demux/27 -> MATLAB Function/33(e27)
  Demux/8 -> MATLAB Function/14(e8)
  Demux/11 -> MATLAB Function/17(e11)
  Demux/7 -> MATLAB Function/13(e7)
  Demux/10 -> MATLAB Function/16(e10)
  Demux/9 -> MATLAB Function/15(e9)
  Demux/22 -> MATLAB Function/28(e22)
  Demux/25 -> MATLAB Function/31(e25)
  Demux/5 -> MATLAB Function/11(e5)
  Demux/23 -> MATLAB Function/29(e23)
  Demux/28 -> MATLAB Function/34(e28)
  Demux/6 -> MATLAB Function/12(e6)
  Demux/12 -> MATLAB Function/18(e12)
  Demux/21 -> MATLAB Function/27(e21)
  Demux/20 -> MATLAB Function/26(e20)
  Demux/18 -> MATLAB Function/24(e18)
  Demux/13 -> MATLAB Function/19(e13)
  Demux/14 -> MATLAB Function/20(e14)
  Demux/19 -> MATLAB Function/25(e19)
  Demux/15 -> MATLAB Function/21(e15)
  Demux/16 -> MATLAB Function/22(e16)
  Demux/17 -> MATLAB Function/23(e17)
  Interpreted MATLAB Function1/1 -> Demux/1
  MATLAB Function/6(t6) -> Out6/1
  MATLAB Function/7(t7) -> Out7/1
  z/1 -> MATLAB Function/3(x3)
  MATLAB Function/5(t5) -> Out5/1
  MATLAB Function/4(t4) -> Out4/1
  MATLAB Function/1(t1) -> Out1/1
  y/1 -> MATLAB Function/2(x2)
  MATLAB Function/3(t3) -> Out3/1
  MATLAB Function/2(t2) -> Out2/1
  x/1 -> MATLAB Function/1(x1)

== system LBR7_Duobot_ResolvedMotion/KUKA LBR 7 iiwa/iiwa_link_0 ==
  Inertia : sm_lib/Body Elements/Solid  InertiaType=Custom  Mass=5  MassUnits=kg  CenterOfMass=[0, 0, 0]  CenterOfMassUnits=m  MomentsOfInertia=[0.05, 0.06, 0.03]  MomentsOfInertiaUnits=kg*m^2  ProductsOfInertia=[0, 0, 0]  ProductsOfInertiaUnits=kg*m^2  DensityBased=on  Density=1000  DensityUnits=kg/m^3  DoExposeReferenceFrame=on  SerializedFrames=<Frames/>  GraphicType=None  MarkerShape=Sphere  MarkerSize=10  GraphicVisPropType=SimpleVisualProperties  GraphicDiffuseColor=[0.5 0.5 0.5]  GraphicSpecularColor=[0.5 0.5 0.5 1.0]  GraphicAmbientColor=[0.15 0.15 0.15 1.0]  GraphicEmissiveColor=[0.0 0.0 0.0 1.0]  GraphicShininess=75  GraphicOpacity=1.0  GeometryShape=Sphere  RectangleSize=[1 1]  RectangleSizeUnits=m  BrickDimensions=[1 1 1]  BrickDimensionUnits=m  CylinderRadius=1  CylinderRadiusUnits=m  CylinderLength=1  CylinderLengthUnits=m  SphereRadius=1  SphereRadiusUnits=m  EllipsoidRadii=[1 1 1]  EllipsoidRadiiUnits=m  ExtrusionCrossSection=[1 1; -1 1; -1 -1; 1 -1]  ExtrusionCrossSectionUnits=m  ExtrusionLength=1  ExtrusionLengthUnits=m  PolygonNumSides=3  PolygonOuterRadius=1  PolygonOuterRadiusUnits=m  ExtGeomFileType=STEP  ExtGeomFileUnits=m  RevolutionCrossSection=[1 1; 1 -1; 2 -1; 2 1]  RevolutionCrossSectionUnits=m  RevolutionExtent=Full  RevolutionAngle=180  RevolutionAngleUnits=deg
  InertiaOriginTransform : sm_lib/Frames and Transforms/Rigid Transform  TranslationMethod=Cartesian  TranslationStandardOffset=0  TranslationLengthUnit=m  TranslationStandardAxis=+Z  TranslationCartesianOffset=[-0.1, 0, 0.07000000000000001]  TranslationROffset=0  TranslationROffsetUnits=m  TranslationZOffset=0  TranslationZOffsetUnits=m  TranslationThetaOffset=0  TranslationThetaOffsetUnits=deg  RotationMethod=RotationSequence  RotationAngleUnits=deg  RotationStandardAxis=+Z  RotationAngle=0.0  RotationArbitraryAxis=[0 0 1]  FollAlignAxisA=+X  BaseAlignAxisA=+Y  FollAlignAxisB=+Y  BaseAlignAxisB=+Z  RotationSequenceAxes=BaseAxes  RotationSequence=XYZ  RotationSequenceAngles=[0, 0, 0]  RotationSequenceAnglesUnits=rad  RotationMatrix=[1 0 0; 0 1 0; 0 0 1]
  ReferenceFrame : sm_lib/Frames and Transforms/Reference Frame
  Visual : sm_lib/Body Elements/Solid  InertiaType=Custom  Mass=0  MassUnits=kg  CenterOfMass=[0, 0, 0]  CenterOfMassUnits=m  MomentsOfInertia=[0, 0, 0]  MomentsOfInertiaUnits=kg*m^2  ProductsOfInertia=[0, 0, 0]  ProductsOfInertiaUnits=kg*m^2  DensityBased=on  Density=1000  DensityUnits=kg/m^3  DoExposeReferenceFrame=on  SerializedFrames=<Frames/>  GraphicType=FromGeometry  MarkerShape=Sphere  MarkerSize=10  GraphicVisPropType=SimpleVisualProperties  GraphicDiffuseColor=[0.4, 0.4, 0.4]  GraphicSpecularColor=[0.5 0.5 0.5 1.0]  GraphicAmbientColor=[0.15 0.15 0.15 1.0]  GraphicEmissiveColor=[0.0 0.0 0.0 1.0]  GraphicShininess=75  GraphicOpacity=1  GeometryShape=FromFile  RectangleSize=[1 1]  RectangleSizeUnits=m  BrickDimensions=[1 1 1]  BrickDimensionUnits=m  CylinderRadius=1  CylinderRadiusUnits=m  CylinderLength=1  CylinderLengthUnits=m  SphereRadius=1  SphereRadiusUnits=m  EllipsoidRadii=[1 1 1]  EllipsoidRadiiUnits=m  ExtrusionCrossSection=[1 1; -1 1; -1 -1; 1 -1]  ExtrusionCrossSectionUnits=m  ExtrusionLength=1  ExtrusionLengthUnits=m  PolygonNumSides=3  PolygonOuterRadius=1  PolygonOuterRadiusUnits=m  ExtGeomFileType=STL  ExtGeomFileName=base_link.stl  ExtGeomFileUnits=m  RevolutionCrossSection=[1 1; 1 -1; 2 -1; 2 1]  RevolutionCrossSectionUnits=m  RevolutionExtent=Full  RevolutionAngle=180  RevolutionAngleUnits=deg
  VisualOriginTransform : sm_lib/Frames and Transforms/Rigid Transform  TranslationMethod=Cartesian  TranslationStandardOffset=0  TranslationLengthUnit=m  TranslationStandardAxis=+Z  TranslationCartesianOffset=[0, 0, 0]  TranslationROffset=0  TranslationROffsetUnits=m  TranslationZOffset=0  TranslationZOffsetUnits=m  TranslationThetaOffset=0  TranslationThetaOffsetUnits=deg  RotationMethod=RotationSequence  RotationAngleUnits=deg  RotationStandardAxis=+Z  RotationAngle=0.0  RotationArbitraryAxis=[0 0 1]  FollAlignAxisA=+X  BaseAlignAxisA=+Y  FollAlignAxisB=+Y  BaseAlignAxisB=+Z  RotationSequenceAxes=BaseAxes  RotationSequence=XYZ  RotationSequenceAngles=[0, 0, 0]  RotationSequenceAnglesUnits=rad  RotationMatrix=[1 0 0; 0 1 0; 0 0 1]
  iiwa_joint_1_AxisTransform : sm_lib/Frames and Transforms/Rigid Transform  TranslationMethod=Cartesian  TranslationStandardOffset=0  TranslationLengthUnit=m  TranslationStandardAxis=+Z  TranslationCartesianOffset=[0, 0, 0]  TranslationROffset=0  TranslationROffsetUnits=m  TranslationZOffset=0  TranslationZOffsetUnits=m  TranslationThetaOffset=0  TranslationThetaOffsetUnits=deg  RotationMethod=ArbitraryAxis  RotationAngleUnits=rad  RotationStandardAxis=+Z  RotationAngle=0  RotationArbitraryAxis=[1, 0, 0]  FollAlignAxisA=+X  BaseAlignAxisA=+Y  FollAlignAxisB=+Y  BaseAlignAxisB=+Z  RotationSequenceAxes=FollowerAxes  RotationSequence=XYX  RotationSequenceAngles=[0 0 0]  RotationSequenceAnglesUnits=deg  RotationMatrix=[1 0 0; 0 1 0; 0 0 1]
  iiwa_joint_1_OriginTransform : sm_lib/Frames and Transforms/Rigid Transform  TranslationMethod=Cartesian  TranslationStandardOffset=0  TranslationLengthUnit=m  TranslationStandardAxis=+Z  TranslationCartesianOffset=[0, 0, 0.15]  TranslationROffset=0  TranslationROffsetUnits=m  TranslationZOffset=0  TranslationZOffsetUnits=m  TranslationThetaOffset=0  TranslationThetaOffsetUnits=deg  RotationMethod=RotationSequence  RotationAngleUnits=deg  RotationStandardAxis=+Z  RotationAngle=0.0  RotationArbitraryAxis=[0 0 1]  FollAlignAxisA=+X  BaseAlignAxisA=+Y  FollAlignAxisB=+Y  BaseAlignAxisB=+Z  RotationSequenceAxes=BaseAxes  RotationSequence=XYZ  RotationSequenceAngles=[0, 0, 0]  RotationSequenceAnglesUnits=rad  RotationMatrix=[1 0 0; 0 1 0; 0 0 1]
  F : PMIOPort  Port=1  Side=Left
  F1 : PMIOPort  Port=2  Side=Right
  connections:
  Inertia/RConn1 -- InertiaOriginTransform/RConn1
  ReferenceFrame/RConn1 -- InertiaOriginTransform/LConn1 -- VisualOriginTransform/LConn1 -- iiwa_joint_1_OriginTransform/LConn1 -- F/RConn1
  Visual/RConn1 -- VisualOriginTransform/RConn1
  iiwa_joint_1_AxisTransform/RConn1 -- F1/RConn1
  iiwa_joint_1_AxisTransform/LConn1 -- iiwa_joint_1_OriginTransform/RConn1
